simulink model "modelClosedLoop_v2"  (R2019b)
settings: Solver=VariableStepAuto  StartTime=0.0  StopTime=Tsim  RelTol=1e-3
values from neighbouring files (symbols this model uses):
  params = load(fullfile(proj_root, 'Planta', 'params', 'param_MF6713.mat'))    [init_sim.m]
  Ts_guidance = 0.05    [init_sim.m]
  useCourse = 1    [init_sim.m]
  vx = 3.5    [init_sim.m]
  wps = resample_waypoints(wps_original, wpDistance)    [init_sim.m]
  X0 = zeros(7, 1)    [init_sim.m]
undefined symbols (not defined in the file or in its folder): Controlador, controllerGainsCurve, userParameters
settings Model: Creator=renan  LastModifiedBy=renan

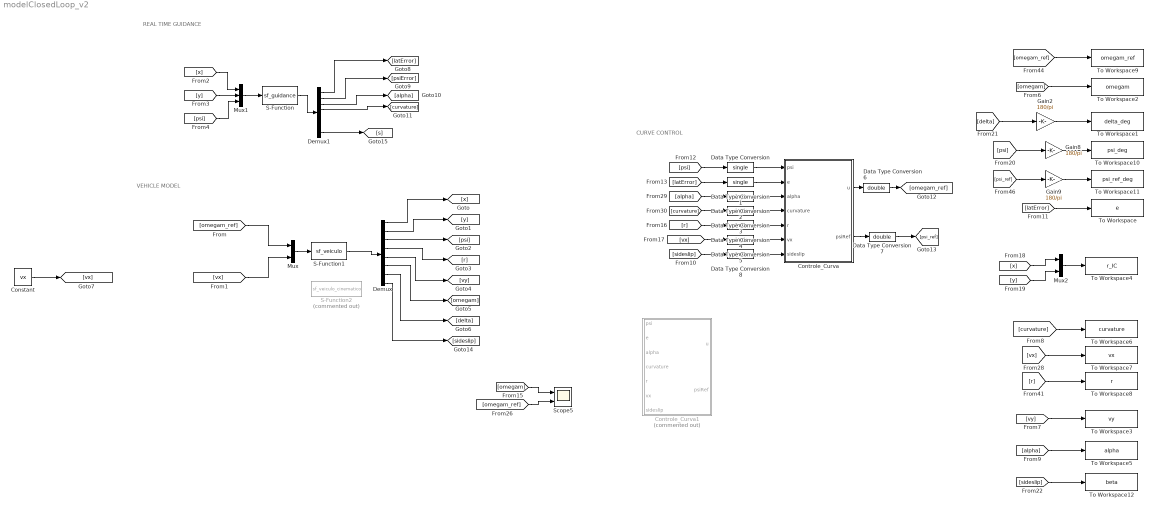
== system modelClosedLoop_v2 ==
  note: CURVE CONTROL
  note: VEHICLE MODEL
  note: REAL TIME GUIDANCE
  Constant : Constant  Value=vx
  Controle_Curva : Subsystem  TreatAsAtomicUnit=on
  Controle_Curva1 : Subsystem  Commented=on  TreatAsAtomicUnit=on
  Data Type Conversion{,1..5,8} (7 alike) : DataTypeConversion  OutDataTypeStr=single
  Data Type Conversion6 : DataTypeConversion  OutDataTypeStr=double
  Data Type Conversion7 : DataTypeConversion  OutDataTypeStr=double
  Demux : Demux  Outputs=8
  Demux1 : Demux  Outputs=8
  Gain2 : Gain  Gain=180/pi
  Gain8 : Gain  Gain=180/pi
  Gain9 : Gain  Gain=180/pi
  Mux : Mux  Inputs=2
  Mux1 : Mux  Inputs=3
  Mux2 : Mux  Inputs=2
  S-Function : S-Function  FunctionName=sf_guidance  Parameters=wps,Ts_guidance  SFunctionDeploymentMode=off  EnableBusSupport=off
  S-Function1 : S-Function  FunctionName=sf_veiculo  Parameters=X0,params  SFunctionDeploymentMode=off  EnableBusSupport=off
  S-Function2 : S-Function  Commented=on  FunctionName=sf_veiculo_cinematico  Parameters=X0,params  SFunctionDeploymentMode=off  EnableBusSupport=off
  Scope5 : Scope  NumInputPorts=2
  To Workspace : ToWorkspace  VariableName=e  SaveFormat=Structure With Time  SampleTime=0.01
  To Workspace1 : ToWorkspace  VariableName=delta_deg  SaveFormat=Structure With Time  SampleTime=0.01
  To Workspace10 : ToWorkspace  VariableName=psi_deg  SaveFormat=Structure With Time  SampleTime=0.01
  To Workspace11 : ToWorkspace  VariableName=psi_ref_deg  SaveFormat=Structure With Time  SampleTime=0.01
  To Workspace12 : ToWorkspace  VariableName=beta  SaveFormat=Structure With Time  SampleTime=0.01
  To Workspace2 : ToWorkspace  VariableName=omegam  SaveFormat=Structure With Time  SampleTime=0.01
  To Workspace3 : ToWorkspace  VariableName=vy  SaveFormat=Structure With Time  SampleTime=0.01
  To Workspace4 : ToWorkspace  VariableName=r_IC  SaveFormat=Structure With Time  SampleTime=0.01
  To Workspace5 : ToWorkspace  VariableName=alpha  SaveFormat=Structure With Time  SampleTime=0.01
  To Workspace6 : ToWorkspace  VariableName=curvature  SaveFormat=Structure With Time  SampleTime=0.01
  To Workspace7 : ToWorkspace  VariableName=vx  SaveFormat=Structure With Time  SampleTime=0.01
  To Workspace8 : ToWorkspace  VariableName=r  SaveFormat=Structure With Time  SampleTime=0.01
  To Workspace9 : ToWorkspace  VariableName=omegam_ref  SaveFormat=Structure With Time  SampleTime=0.01
  wires:
  Mux/1 -> S-Function1/1
  [omegam_ref] -> Mux/1
  [vx] -> Mux/2
  S-Function1/1 -> Demux/1
  Demux/1 -> [x]
  Demux/2 -> [y]
  Demux/3 -> [psi]
  Demux/4 -> [r]
  Demux/5 -> [vy]
  Demux/6 -> [omegam]
  Demux/7 -> [delta]
  Constant/1 -> [vx]
  [x] -> Mux1/1
  [y] -> Mux1/2
  Mux1/1 -> S-Function/1
  [psi] -> Mux1/3
  S-Function/1 -> Demux1/1
  Demux1/1 -> [latError]
  Demux1/2 -> [psiError]
  Demux1/3 -> [alpha]
  Demux1/4 -> [curvature]
  [latError] -> Data Type Conversion1/1
  [r] -> Data Type Conversion4/1
  [vx] -> Data Type Conversion5/1
  Controle_Curva/1(u) -> Data Type Conversion6/1
  Data Type Conversion/1 -> Controle_Curva/1(psi)
  Data Type Conversion1/1 -> Controle_Curva/2(e)
  Data Type Conversion2/1 -> Controle_Curva/3(alpha)
  Data Type Conversion3/1 -> Controle_Curva/4(curvature)
  Data Type Conversion4/1 -> Controle_Curva/5(r)
  Data Type Conversion5/1 -> Controle_Curva/6(vx)
  Data Type Conversion6/1 -> [omegam_ref]
  [curvature] -> To Workspace6/1
  Gain8/1 -> To Workspace10/1
  [latError] -> To Workspace/1
  [psi] -> Gain8/1
  Gain2/1 -> To Workspace1/1
  Gain9/1 -> To Workspace11/1
  [psi_ref] -> Gain9/1
  [omegam] -> To Workspace2/1
  [r] -> To Workspace8/1
  [omegam_ref] -> To Workspace9/1
  [vx] -> To Workspace7/1
  Mux2/1 -> To Workspace4/1
  [delta] -> Gain2/1
  Controle_Curva/2(psiRef) -> Data Type Conversion7/1
  Data Type Conversion7/1 -> [psi_ref]
  [x] -> Mux2/1
  [y] -> Mux2/2
  [vy] -> To Workspace3/1
  [alpha] -> To Workspace5/1
  Demux/8 -> [sideslip]
  [psi] -> Data Type Conversion/1
  [sideslip] -> Data Type Conversion8/1
  Data Type Conversion8/1 -> Controle_Curva/7(sideslip)
  [sideslip] -> To Workspace12/1
  Demux1/8 -> [s]
  [omegam] -> Scope5/1
  [omegam_ref] -> Scope5/2
  [alpha] -> Data Type Conversion2/1
  [curvature] -> Data Type Conversion3/1

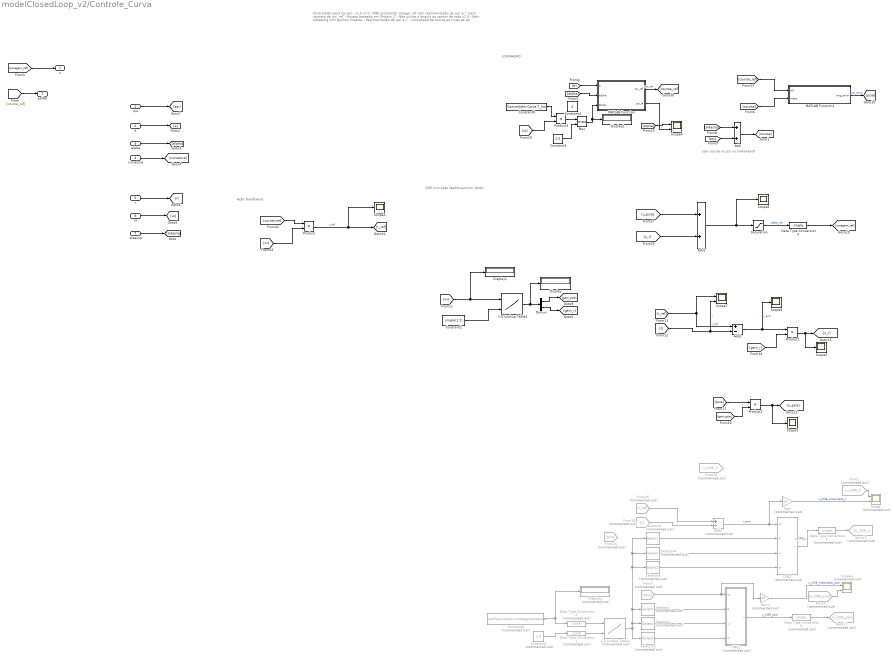
== system modelClosedLoop_v2/Controle_Curva ==
  note: usar course ou psi no lookahead?
  note: Controlador para Curvas - v2.0
      |
      | v1.0
      | - CME calculando 'omega_ref' com realimentação de 'psi' e 'r' para rastreio de 'psi_ref'
      | - Projeto baseado em 'Projeto_2'
      | - Não utiliza o ângulo do sensor de roda
      |
      | v2.0
      | - Gain schedulig com ganhos lineares
      | - Realimentação de 'psi' e 'r'
      | - Lookahead de course ao invés de psi
  note: LOOKAHEAD
  note: CME com ação feedfoward em 'delta'
  note: Ação feedfoward
  psi : Inport  OutDataTypeStr=single  PortDimensions=1
  e : Inport  Port=2  OutDataTypeStr=single  PortDimensions=1
  alpha : Inport  Port=3  OutDataTypeStr=single  PortDimensions=1
  curvature : Inport  Port=4  OutDataTypeStr=single  PortDimensions=1
  r : Inport  Port=5  OutDataTypeStr=single  PortDimensions=1
  vx : Inport  Port=6  OutDataTypeStr=single  PortDimensions=1
  sideslip : Inport  Port=7
  1-D Lookup Table1 : Lookup_n-D  Commented=on  BreakpointsForDimension1=uint8(1:7)  BreakpointsForDimension2=uint8(1:8)  IndexSearchMethod=Linear search  BeginIndexSearchUsingPreviousIndexResult=on  Table=controllerGainsCurve  ExtrapMethod=Clip  UseLastTableValue=on  InternalRulePriority=Speed  OutDataTypeStr=single  RndMeth=Simplest  InputSameDT=on
  1-D Lookup Table2 : Lookup_n-D  BreakpointsForDimension1=Controlador.Curva.v_index  BreakpointsForDimension2=uint8(1:2)  IndexSearchMethod=Linear search  BeginIndexSearchUsingPreviousIndexResult=on  Table=Controlador.Curva.Gains  ExtrapMethod=Clip  UseLastTableValue=on  InternalRulePriority=Speed  OutDataTypeStr=single  RndMeth=Simplest  InputSameDT=on
  Add : Sum
  Add1 : Sum
  Add2 : Sum  Inputs=+-
  Add3 : Sum  Commented=on  Inputs=+-
  CME1 : MATLAB Function  Commented=on  TreatAsAtomicUnit=on
  CME2 : MATLAB Function  Commented=on  TreatAsAtomicUnit=on
  Constant1 : Constant  Commented=on  Value=1:8
  Constant2 : Constant  Value=single(1:2)
  Constant3 : Constant  Value=2.0
  Constant4 : Constant  Value=4
  Constant6 : Constant  Commented=on  Value=userParameters.curveAggressiveness
  Constant8 : Constant  Value=Controlador.Curva.T_look  SampleTime=-1
  Data Type Conversion1 : DataTypeConversion  Commented=on  OutDataTypeStr=uint8
  Data Type Conversion2 : DataTypeConversion  Commented=on  OutDataTypeStr=uint8
  Data Type Conversion3 : DataTypeConversion  OutDataTypeStr=single
  Data Type Conversion8 : DataTypeConversion  Commented=on  OutDataTypeStr=single
  Data Type Conversion9 : DataTypeConversion  Commented=on  OutDataTypeStr=single
  Demux : Demux  Outputs=2
  Display : Display
  Display1 : Display
  Display2 : Display
  Display4 : Display  Commented=on
  From15 : From  Commented=on  GotoTag=psie
  From16 : From  Commented=on  GotoTag=r
  From2 : From  Commented=on  GotoTag=u_CME_r
  From20 : From  Commented=on  GotoTag=u_CME_r
  From26 : From  Commented=on  GotoTag=r_ref
  From3 : From  Commented=on  GotoTag=u_CME_psie
  From7 : From  Commented=on  GotoTag=psie
  Gain : Gain  Commented=on  Gain=52
  Gain1 : Gain  Commented=on  Gain=43
  Goto11 : Goto  Commented=on  GotoTag=u_CME_psie
  Goto15 : Goto  Commented=on  GotoTag=u_CME_r
  MATLAB Function : MATLAB Function  TreatAsAtomicUnit=on
  MATLAB Function1 : MATLAB Function  TreatAsAtomicUnit=on
  Max : MinMax  Function=max  Inputs=2
  Product{,1..3} (4 alike) : Product
  Saturation : Saturate  UpperLimit=Controlador.Curva.omegam_sat  LowerLimit=-Controlador.Curva.omegam_sat
  Scope : Scope  Commented=on  NumInputPorts=2
  Scope1 : Scope  Commented=on  NumInputPorts=2
  Scope{2..3,5,8..9} (5 alike) : Scope
  Scope4 : Scope  NumInputPorts=2
  Scope7 : Scope  NumInputPorts=2
  Selector : Selector  Commented=on  InputPortWidth=8  IndexOptions=Index vector (dialog)  Indices=[2]  OutputSizes=1
  Selector1 : Selector  Commented=on  InputPortWidth=8  IndexOptions=Index vector (dialog)  Indices=[3 4]  OutputSizes=1
  Selector2 : Selector  Commented=on  InputPortWidth=8  IndexOptions=Index vector (dialog)  Indices=[1]  OutputSizes=1
  Selector3 : Selector  Commented=on  InputPortWidth=8  IndexOptions=Index vector (dialog)  Indices=[6]  OutputSizes=1
  Selector4 : Selector  Commented=on  InputPortWidth=8  IndexOptions=Index vector (dialog)  Indices=[7 8]  OutputSizes=1
  Selector5 : Selector  Commented=on  InputPortWidth=8  IndexOptions=Index vector (dialog)  Indices=[5]  OutputSizes=1
  u : Outport
  psiRef : Outport  Port=2
  wires:
  MATLAB Function1/1(ang_error) -> [psie]  "psi_error"
  [e] -> MATLAB Function/1(e)
  [alpha] -> MATLAB Function/2(alpha)
  Add1/1 -> Scope8/1, Saturation/1
  CME2/1(u) -> Data Type Conversion9/1  "u_CME_r"
  CME1/1(u) -> Data Type Conversion8/1  "u_CME_psie"
  From26/1 -> Add3/1
  From16/1 -> Add3/2
  Product/1 -> Scope5/1, [r_ref]  "r_ref"
  [curvature] -> Product/1
  [vx] -> Product/2
  psi/1 -> [psi]
  e/1 -> [e]
  alpha/1 -> [alpha]
  curvature/1 -> [curvature]
  r/1 -> [r]
  Add3/1 -> Gain/1, CME2/1(et)  "r_erro"
  [omegam_ref] -> u/1
  vx/1 -> [vx]
  From7/1 -> CME1/1(et), Gain1/1
  Selector/1 -> CME1/2(B)
  Selector1/1 -> CME1/3(ur)
  Selector2/1 -> CME1/4(er)
  Selector3/1 -> CME2/2(B)
  Selector4/1 -> CME2/3(ur)
  Selector5/1 -> CME2/4(er)
  Data Type Conversion8/1 -> Goto11/1
  Data Type Conversion9/1 -> Goto15/1
  Gain/1 -> Scope/2  "u_CME_Linearizado_r"
  Gain1/1 -> Scope1/1  "u_CME_linearizado_psie"
  Constant6/1 -> Display4/1, Data Type Conversion2/1
  Constant1/1 -> Data Type Conversion1/1
  1-D Lookup Table1/1 -> Selector3/1, Selector4/1, Selector5/1, Selector/1, Selector1/1, Selector2/1
  Data Type Conversion2/1 -> 1-D Lookup Table1/1
  Data Type Conversion1/1 -> 1-D Lookup Table1/2
  [course_ref] -> psiRef/1
  From2/1 -> Scope/1
  From3/1 -> Scope1/2
  sideslip/1 -> [sideslip]
  [sideslip] -> Add/1
  [psi] -> Add/2
  Add/1 -> [course]
  [vx] -> Display1/1, 1-D Lookup Table2/1
  Constant2/1 -> 1-D Lookup Table2/2
  1-D Lookup Table2/1 -> Display/1, Demux/1
  Demux/1 -> [gain_psie]
  Demux/2 -> [gain_r]
  [r_ref] -> Add2/1, Scope7/1  "r_ref"
  Add2/1 -> Scope9/1, Product1/1  "r_erro"
  [r] -> Scope7/2, Add2/2  "r"
  [psie] -> Product2/1
  Product2/1 -> Scope3/1, [u_psie]
  Product1/1 -> Scope2/1, [u_r]
  Constant8/1 -> Product3/1
  [vx] -> Product3/2
  Product3/1 -> Max/1
  Max/1 -> MATLAB Function/3(Delta), Display2/1
  Constant3/1 -> Max/2
  [u_psie] -> Add1/1
  [u_r] -> Add1/2
  [course] -> MATLAB Function1/2(meas)
  Data Type Conversion3/1 -> [omegam_ref]
  [alpha] -> Scope4/1
  MATLAB Function/2(psi_la) -> Scope4/2
  [course_ref] -> MATLAB Function1/1(ref)
  MATLAB Function/1(psi_ref) -> [course_ref]  "psi_ref"
  [gain_psie] -> Product2/2
  [gain_r] -> Product1/2
  Saturation/1 -> Data Type Conversion3/1  "delta_ref"

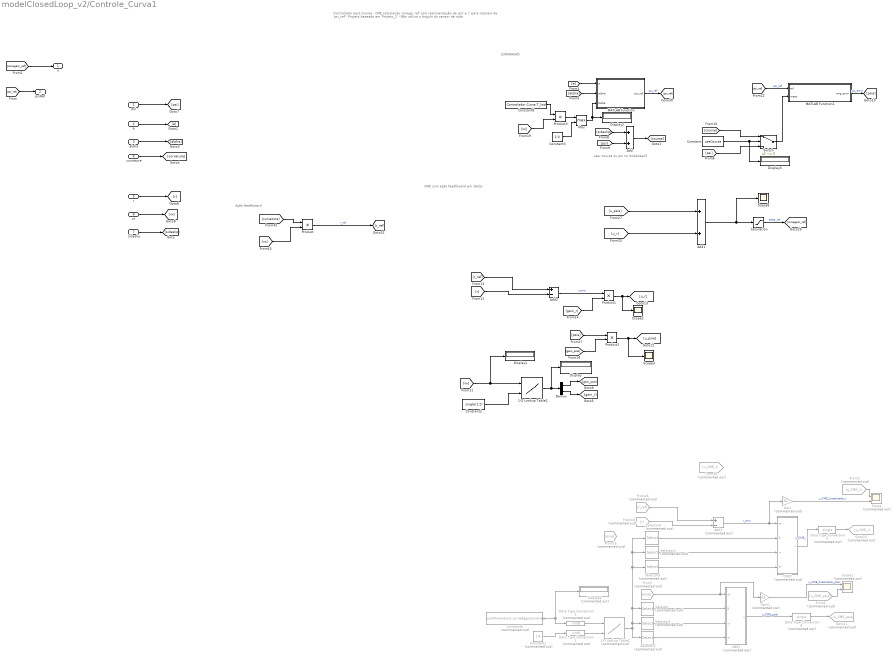
== system modelClosedLoop_v2/Controle_Curva1 ==
  note: Ação feedfoward
  note: CME com ação feedfoward em 'delta'
  note: LOOKAHEAD
  note: Controlador para Curvas
      |
      | - CME calculando 'omega_ref' com realimentação de 'psi' e 'r' para rastreio de 'psi_ref'
      | - Projeto baseado em 'Projeto_2'
      | - Não utiliza o ângulo do sensor de roda
  note: usar course ou psi no lookahead?
  psi : Inport  OutDataTypeStr=single  PortDimensions=1
  e : Inport  Port=2  OutDataTypeStr=single  PortDimensions=1
  alpha : Inport  Port=3  OutDataTypeStr=single  PortDimensions=1
  curvature : Inport  Port=4  OutDataTypeStr=single  PortDimensions=1
  r : Inport  Port=5  OutDataTypeStr=single  PortDimensions=1
  vx : Inport  Port=6  OutDataTypeStr=single  PortDimensions=1
  sideslip : Inport  Port=7
  1-D Lookup Table1 : Lookup_n-D  Commented=on  BreakpointsForDimension1=uint8(1:7)  BreakpointsForDimension2=uint8(1:8)  IndexSearchMethod=Linear search  BeginIndexSearchUsingPreviousIndexResult=on  Table=controllerGainsCurve  ExtrapMethod=Clip  UseLastTableValue=on  InternalRulePriority=Speed  OutDataTypeStr=single  RndMeth=Simplest  InputSameDT=on
  1-D Lookup Table2 : Lookup_n-D  BreakpointsForDimension1=Controlador.Curva.v_index  BreakpointsForDimension2=uint8(1:2)  IndexSearchMethod=Linear search  BeginIndexSearchUsingPreviousIndexResult=on  Table=Controlador.Curva.Gains  ExtrapMethod=Clip  UseLastTableValue=on  InternalRulePriority=Speed  OutDataTypeStr=single  RndMeth=Simplest  InputSameDT=on
  Add : Sum
  Add1 : Sum
  Add2 : Sum  Inputs=+-
  Add3 : Sum  Commented=on  Inputs=+-
  CME1 : MATLAB Function  Commented=on  TreatAsAtomicUnit=on
  CME2 : MATLAB Function  Commented=on  TreatAsAtomicUnit=on
  Constant : Constant  Value=useCourse
  Constant1 : Constant  Commented=on  Value=1:8
  Constant2 : Constant  Value=single(1:2)
  Constant3 : Constant  Value=2.0
  Constant6 : Constant  Commented=on  Value=userParameters.curveAggressiveness
  Constant8 : Constant  Value=Controlador.Curva.T_look  SampleTime=-1
  Data Type Conversion1 : DataTypeConversion  Commented=on  OutDataTypeStr=uint8
  Data Type Conversion2 : DataTypeConversion  Commented=on  OutDataTypeStr=uint8
  Data Type Conversion8 : DataTypeConversion  Commented=on  OutDataTypeStr=single
  Data Type Conversion9 : DataTypeConversion  Commented=on  OutDataTypeStr=single
  Demux : Demux  Outputs=2
  Display{,1..3} (4 alike) : Display
  Display4 : Display  Commented=on
  From15 : From  Commented=on  GotoTag=psie
  From16 : From  Commented=on  GotoTag=r
  From2 : From  Commented=on  GotoTag=u_CME_r
  From20 : From  Commented=on  GotoTag=u_CME_r
  From26 : From  Commented=on  GotoTag=r_ref
  From3 : From  Commented=on  GotoTag=u_CME_psie
  From7 : From  Commented=on  GotoTag=psie
  Gain : Gain  Commented=on  Gain=52
  Gain1 : Gain  Commented=on  Gain=43
  Goto11 : Goto  Commented=on  GotoTag=u_CME_psie
  Goto15 : Goto  Commented=on  GotoTag=u_CME_r
  MATLAB Function : MATLAB Function  TreatAsAtomicUnit=on
  MATLAB Function1 : MATLAB Function  TreatAsAtomicUnit=on
  Max : MinMax  Function=max  Inputs=2
  Product{,1..3} (4 alike) : Product
  Saturation : Saturate  UpperLimit=Controlador.Curva.omegam_sat  LowerLimit=-Controlador.Curva.omegam_sat
  Scope : Scope  Commented=on  NumInputPorts=2
  Scope1 : Scope  Commented=on  NumInputPorts=2
  Scope2 : Scope
  Scope3 : Scope
  Scope8 : Scope
  Selector : Selector  Commented=on  InputPortWidth=8  IndexOptions=Index vector (dialog)  Indices=[2]  OutputSizes=1
  Selector1 : Selector  Commented=on  InputPortWidth=8  IndexOptions=Index vector (dialog)  Indices=[3 4]  OutputSizes=1
  Selector2 : Selector  Commented=on  InputPortWidth=8  IndexOptions=Index vector (dialog)  Indices=[1]  OutputSizes=1
  Selector3 : Selector  Commented=on  InputPortWidth=8  IndexOptions=Index vector (dialog)  Indices=[6]  OutputSizes=1
  Selector4 : Selector  Commented=on  InputPortWidth=8  IndexOptions=Index vector (dialog)  Indices=[7 8]  OutputSizes=1
  Selector5 : Selector  Commented=on  InputPortWidth=8  IndexOptions=Index vector (dialog)  Indices=[5]  OutputSizes=1
  Switch : Switch  Criteria=u2 ~= 0
  u : Outport
  psiRef : Outport  Port=2
  wires:
  [gain_r] -> Product1/2
  [gain_psie] -> Product2/2
  [u_r] -> Add1/2
  [u_psie] -> Add1/1
  Constant3/1 -> Max/2
  Max/1 -> MATLAB Function/3(Delta), Display2/1
  Product3/1 -> Max/1
  [vx] -> Product3/2
  Constant8/1 -> Product3/1
  Product1/1 -> [u_r], Scope2/1
  Product2/1 -> [u_psie], Scope3/1
  [psie] -> Product2/1
  [r] -> Add2/2
  Add2/1 -> Product1/1  "r_erro"
  [r_ref] -> Add2/1
  Demux/2 -> [gain_r]
  Demux/1 -> [gain_psie]
  1-D Lookup Table2/1 -> Demux/1, Display/1
  Constant2/1 -> 1-D Lookup Table2/2
  [vx] -> 1-D Lookup Table2/1, Display1/1
  [psi] -> Switch/3
  [course] -> Switch/1
  Constant/1 -> Switch/2, Display3/1
  Switch/1 -> MATLAB Function1/2(meas)
  Add/1 -> [course]
  [psi] -> Add/2
  [sideslip] -> Add/1
  sideslip/1 -> [sideslip]
  From3/1 -> Scope1/2
  From2/1 -> Scope/1
  [psi_ref] -> psiRef/1
  Data Type Conversion1/1 -> 1-D Lookup Table1/2
  Data Type Conversion2/1 -> 1-D Lookup Table1/1
  1-D Lookup Table1/1 -> Selector2/1, Selector1/1, Selector/1, Selector5/1, Selector4/1, Selector3/1
  Constant1/1 -> Data Type Conversion1/1
  Constant6/1 -> Data Type Conversion2/1, Display4/1
  Gain1/1 -> Scope1/1  "u_CME_linearizado_psie"
  Gain/1 -> Scope/2  "u_CME_Linearizado_r"
  Data Type Conversion9/1 -> Goto15/1
  Data Type Conversion8/1 -> Goto11/1
  Selector5/1 -> CME2/4(er)
  Selector4/1 -> CME2/3(ur)
  Selector3/1 -> CME2/2(B)
  Selector2/1 -> CME1/4(er)
  Selector1/1 -> CME1/3(ur)
  Selector/1 -> CME1/2(B)
  From7/1 -> Gain1/1, CME1/1(et)
  vx/1 -> [vx]
  [omegam_ref] -> u/1
  Add3/1 -> CME2/1(et), Gain/1  "r_erro"
  r/1 -> [r]
  curvature/1 -> [curvature]
  alpha/1 -> [alpha]
  e/1 -> [e]
  psi/1 -> [psi]
  [vx] -> Product/2
  [curvature] -> Product/1
  Product/1 -> [r_ref]  "r_ref"
  Saturation/1 -> [omegam_ref]  "delta_ref"
  From16/1 -> Add3/2
  From26/1 -> Add3/1
  CME1/1(u) -> Data Type Conversion8/1  "u_CME_psie"
  CME2/1(u) -> Data Type Conversion9/1  "u_CME_r"
  Add1/1 -> Saturation/1, Scope8/1
  [alpha] -> MATLAB Function/2(alpha)
  [e] -> MATLAB Function/1(e)
  MATLAB Function1/1(ang_error) -> [psie]  "psi_error"
  MATLAB Function/1(psi_ref) -> [psi_ref]  "psi_ref"
  [psi_ref] -> MATLAB Function1/1(ref)  "psi_ref"

== matlab function modelClosedLoop_v2/Controle_Curva1/CME1 ==
  data: u output size=1; et input size=1; B input size=1; ur input size=[2,1]; er input size=1
% et: erro (ref-meas)
% B: Parâmetro 3
% ur: Parâmetro 2 (batentes do controle)
% er: Parâmetro
function u = CME(et, B, ur, er)


umin = ur(1); umax = ur(2);
% Cálculo do erro
%et = yref - y;
e = et / er;
if e < -1, e = single(-1);  elseif e > 1, e = single(1); end
% Cálculo de u
if abs(e) == 1, ut = e; else ss = e - sign(e); ut = sign(ss) * (abs(ss) ^ (2 ^ -B) - 1); end
% Cálculo da saída
a = (umax - umin) / 2; u = a * (ut - 1) + umax;

end

== matlab function modelClosedLoop_v2/Controle_Curva/MATLAB Function ==
  data: e input; psi_ref output; alpha input; Delta input; psi_la output
function [psi_ref, psi_la] = Lookahead(e, alpha, Delta)

psi_la = atan(-e/Delta);
psi_ref = alpha + atan(-e/Delta);

== matlab function modelClosedLoop_v2/Controle_Curva/MATLAB Function1 ==
  data: ref input; ang_error output; meas input
% ref-meas
function ang_error = Angular_Error(ref, meas)

    ref = mod(ref, 2*pi);
    meas = mod(meas, 2*pi);
    
    if(meas > ref)
        if(abs(2*pi-meas+ref) < abs(ref-meas))
            ang_error = 2*pi-meas+ref;
        else
            ang_error = ref - meas;
        end
    elseif (meas < ref)
        if(abs(meas - ref) < abs(2*pi-ref+meas))
            ang_error = ref - meas;
        else
            ang_error = -(meas + 2*pi - ref);
        end
    else
        ang_error = single(0);
    end
end

== matlab function modelClosedLoop_v2/Controle_Curva/CME1 ==
  data: u output size=1; et input size=1; B input size=1; ur input size=[2,1]; er input size=1
% et: erro (ref-meas)
% B: Parâmetro 3
% ur: Parâmetro 2 (batentes do controle)
% er: Parâmetro
function u = CME(et, B, ur, er)


umin = ur(1); umax = ur(2);
% Cálculo do erro
%et = yref - y;
e = et / er;
if e < -1, e = single(-1);  elseif e > 1, e = single(1); end
% Cálculo de u
if abs(e) == 1, ut = e; else ss = e - sign(e); ut = sign(ss) * (abs(ss) ^ (2 ^ -B) - 1); end
% Cálculo da saída
a = (umax - umin) / 2; u = a * (ut - 1) + umax;

end

== matlab function modelClosedLoop_v2/Controle_Curva1/CME2 ==
  data: u output size=1; et input size=1; B input size=1; ur input size=[2,1]; er input size=1
% et: erro (ref-meas)
% B: Parâmetro 3
% ur: Parâmetro 2 (batentes do controle)
% er: Parâmetro
function u = CME(et, B, ur, er)


umin = ur(1); umax = ur(2);
% Cálculo do erro
%et = yref - y;

e = et / er;

if e < -1
    e = single(-1);
elseif e > 1
    e = single(1);
end

% Cálculo de u
if abs(e) == 1
    ut = e;
else
    ss = e - sign(e);
    ut = sign(ss) * (abs(ss) ^ (2 ^ -B) - 1);
end

% Cálculo da saída
a = (umax - umin) / 2; u = a * (ut - 1) + umax;

end

== matlab function modelClosedLoop_v2/Controle_Curva/CME2 ==
  data: u output size=1; et input size=1; B input size=1; ur input size=[2,1]; er input size=1
% et: erro (ref-meas)
% B: Parâmetro 3
% ur: Parâmetro 2 (batentes do controle)
% er: Parâmetro
function u = CME(et, B, ur, er)


umin = ur(1); umax = ur(2);
% Cálculo do erro
%et = yref - y;

e = et / er;

if e < -1
    e = single(-1);
elseif e > 1
    e = single(1);
end

% Cálculo de u
if abs(e) == 1
    ut = e;
else
    ss = e - sign(e);
    ut = sign(ss) * (abs(ss) ^ (2 ^ -B) - 1);
end

% Cálculo da saída
a = (umax - umin) / 2; u = a * (ut - 1) + umax;

end

== matlab function modelClosedLoop_v2/Controle_Curva1/MATLAB Function ==
  data: e input; psi_ref output; alpha input; Delta input
function psi_ref = Lookahead(e, alpha, Delta)

psi_ref = alpha + atan(-e/Delta);

== matlab function modelClosedLoop_v2/Controle_Curva1/MATLAB Function1 ==
  data: ref input; ang_error output; meas input
% ref-meas
function ang_error = Angular_Error(ref, meas)

    ref = mod(ref, 2*pi);
    meas = mod(meas, 2*pi);
    
    if(meas > ref)
        if(abs(2*pi-meas+ref) < abs(ref-meas))
            ang_error = 2*pi-meas+ref;
        else
            ang_error = ref - meas;
        end
    elseif (meas < ref)
        if(abs(meas - ref) < abs(2*pi-ref+meas))
            ang_error = ref - meas;
        else
            ang_error = -(meas + 2*pi - ref);
        end
    else
        ang_error = single(0);
    end
end
